simulink model "DC_motor_simulink"  (R2024b)
settings: Solver=ode45  StartTime=0.0  StopTime=2000  RelTol=1e-3
model workspace (MAT data in the model file):
  S = [0; 0; 0.05; 0; 0; -0.05; 0; 0]
values from neighbouring files (symbols this model uses):
  B = 0.81    [DC_motor_script.m]
  d = 680e-3    (= 0.68)    [DC_motor_script.m]
  E_n = Ks*Ie_r*omega_b    (= 538.36426107)    [DC_motor_script.m]
  Ie_r = 5    [DC_motor_script.m]
  J = m_max*((rho^2*d^2)/4)    (= 90.6180715851)    [DC_motor_script.m]
  Ks = 1.06    [DC_motor_script.m]
  L = [0;1;3;4;6;8;9;10]    [DC_motor_script.m]
  La = tau_a*Ra    (= 0.0039)    [DC_motor_script.m]
  Le = tau_e*Re    (= 1.2)    [DC_motor_script.m]
  m_max = mt+130*80    (= 25400)    [DC_motor_script.m]
  omega_b = 970*(2*pi/60)    (= 101.578162466)    [DC_motor_script.m]
  omega_max = (v_max/3.6)*2/(d*rho)    (= 195.32428356)    [DC_motor_script.m]
  Ra = 0.39    [DC_motor_script.m]
  Re = 12    [DC_motor_script.m]
  rho = 13/74    (= 0.175675675676)    [DC_motor_script.m]
  Tn = Pr_tot/omega_b    (= 826.949395034)    [DC_motor_script.m]
  V = [v_r/2;v_r;v_r;v_max;v_r;v_r;v_r/2;0]    [DC_motor_script.m]
  Va_r = 600    [DC_motor_script.m]
  Ve_r = 60    [DC_motor_script.m]
undefined symbols (not defined in the file or in its folder): Ccurr, Cexc_curr, Cspeed
libraries: slpidlib x3
settings Model: Creator=migli  LastModifiedBy=migli

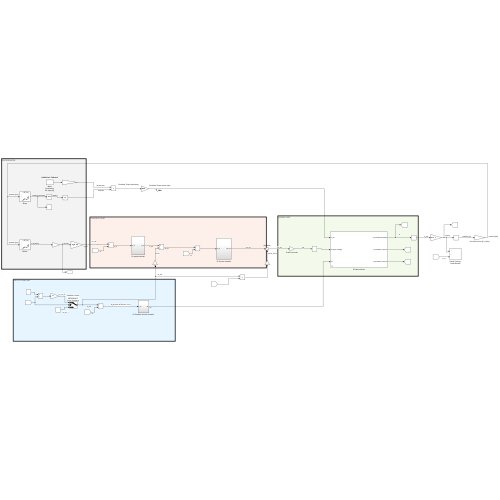
[thumbnail: Simulink's stored preview of the top-level diagram]
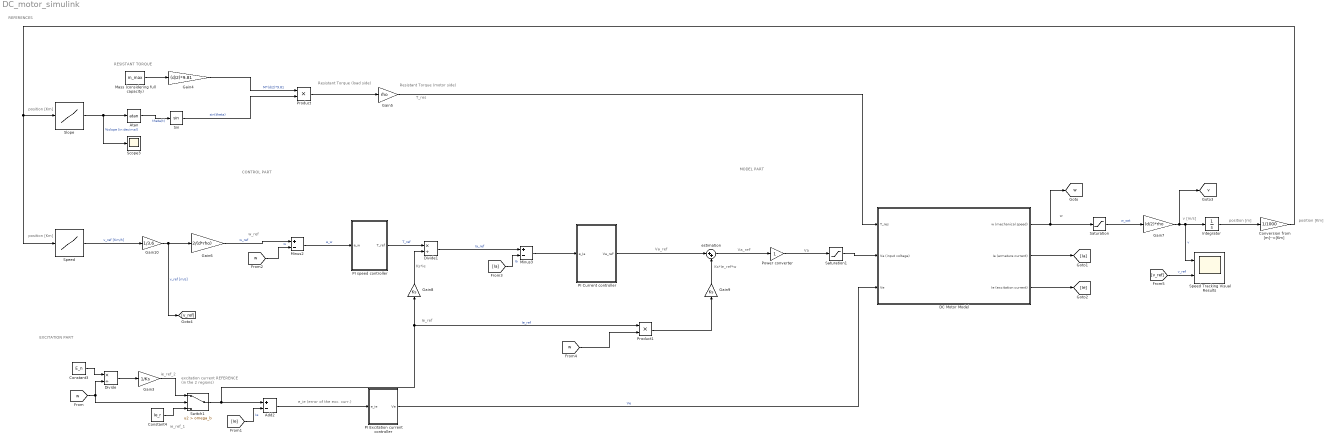
== system DC_motor_simulink ==
  note: T_res
  note: MODEL PART
  note: REFERENCES
  note: CONTROL PART
  note: EXCITATION PART
  note: position [m]
  note: e_ie (error of the exc. curr.)
  note: Va
  note: Va_ref'
  note: Va_ref
  note: Ks*ie
  note: position [Km]
  note: RESISTANT TORQUE
  note: Resistant Torque (motor side)
  note: Resistant Torque (load side)
  note: w_ref
  note: position [Km]
  note: excitation current
      |   REFERENCE
      | (in the 2 regions)
  note: ie_ref_2
  note: ie_ref_1
  note: Ie_ref
  note: Ks*Ie_ref*w
  note: position [Km]
  note: v [m/s]
  note: w
  Add2 : Sum  Inputs=+-
  Atan : Trigonometry  Operator=atan
  Constant3 : Constant  Value=E_n
  Constant4 : Constant  Value=Ie_r
  "Conversion from [m]-->[Km] " : Gain  Gain=1/1000
  DC Motor Model : Subsystem
      mask DialogControl DescTextVar Prompt: PMDC model
  Divide : Product  Inputs=*/
  Divide1 : Product  Inputs=*/
  Gain10 : Gain  Gain=1/3.6
  Gain3 : Gain  Gain=1/Ks
  Gain4 : Gain  Gain=(d/2)*9.81
  Gain5 : Gain  Gain=rho
  Gain6 : Gain  Gain=2/(d*rho)
  Gain7 : Gain  Gain=(d/2)*rho
  Gain8 : Gain  Gain=Ks
  Gain9 : Gain  Gain=Ks
  Integrator : Integrator
  Mass (considering full capacity) : Constant  Value=m_max
  Minus2 : Sum  Inputs=+-
  Minus3 : Sum  Inputs=+-
  PI Current controller : Subsystem
  PI Excitation current controller : Subsystem
  PI speed controller : Subsystem
  Power converter : Gain
  Product : Product
  Product1 : Product
  Saturation : Saturate  UpperLimit=omega_max+300  LowerLimit=0
  Saturation1 : Saturate  UpperLimit=Va_r*1000  LowerLimit=-Va_r*1000
  Scope3 : Scope
  Sin : Trigonometry
  Slope : Lookup_n-D  NumberOfTableDimensions=1  BreakpointsForDimension1=L  Table=S  InterpMethod=Flat  InternalRulePriority=Speed  RndMeth=Simplest
  Speed : Lookup_n-D  NumberOfTableDimensions=1  BreakpointsForDimension1=L  Table=V  InterpMethod=Flat  InternalRulePriority=Speed  RndMeth=Simplest
  Speed Tracking Visual Results : Scope  NumInputPorts=2
  Switch1 : Switch  Criteria=u2 > Threshold  Threshold=omega_b  SaturateOnIntegerOverflow=off  InputSameDT=off
  estimation : Sum  Inputs=|++
  tag scope: v=global, w=global
  wires:
  Atan/1 -> Sin/1  "theta(t)"
  Mass (considering full capacity)/1 -> Gain4/1
  Product/1 -> Gain5/1
  Slope/1 -> Scope3/1, Atan/1  "%slope (in decimal)"
  Sin/1 -> Product/2  "sin(theta)"
  Gain4/1 -> Product/1  "M*(d/2)*9.81"
  Speed/1 -> Gain10/1  "v_ref [Km/h]"
  Gain6/1 -> Minus2/1  "w_ref"
  [w] -> Minus2/2  "w"
  Minus2/1 -> PI speed controller/1(e_w)  "e_w"
  PI speed controller/1(T_ref) -> Divide1/1  "T_ref"
  Gain8/1 -> Divide1/2
  Gain3/1 -> Switch1/1
  Constant4/1 -> Switch1/3
  [w] -> Divide/2, Switch1/2
  Switch1/1 -> Product1/1, Gain8/1, Add2/1  "Ie_ref"
  [Ie] -> Add2/2  "Ie"
  Constant3/1 -> Divide/1
  Divide/1 -> Gain3/1
  Divide1/1 -> Minus3/1  "Ia_ref"
  [Ia] -> Minus3/2  "Ia"
  Minus3/1 -> PI Current controller/1(e_Ia)
  PI Current controller/1(Va_ref') -> estimation/1
  Gain9/1 -> estimation/2
  [w] -> Product1/2
  Product1/1 -> Gain9/1
  estimation/1 -> Power converter/1
  Power converter/1 -> Saturation1/1
  Saturation1/1 -> DC Motor Model/2(Va (input voltage))
  Gain5/1 -> DC Motor Model/1(T_res)
  Add2/1 -> PI Excitation current controller/1(e_ie)
  PI Excitation current controller/1(Ve) -> DC Motor Model/3(Ve)  "Ve"
  Gain7/1 -> [v], Speed Tracking Visual Results/1, Integrator/1  "v"
  Integrator/1 -> "Conversion from [m]-->[Km] "/1
  "Conversion from [m]-->[Km] "/1 -> Speed/1, Slope/1
  DC Motor Model/2(Ia (armature current)) -> [Ia]
  DC Motor Model/3(Ie (excitation current)) -> [Ie]
  Gain10/1 -> [v_ref], Gain6/1  "v_ref [m/s]"
  DC Motor Model/1(w (mechanical speed)) -> [w], Saturation/1
  Saturation/1 -> Gain7/1  "w_sat"
  [v_ref] -> Speed Tracking Visual Results/2  "v_ref"

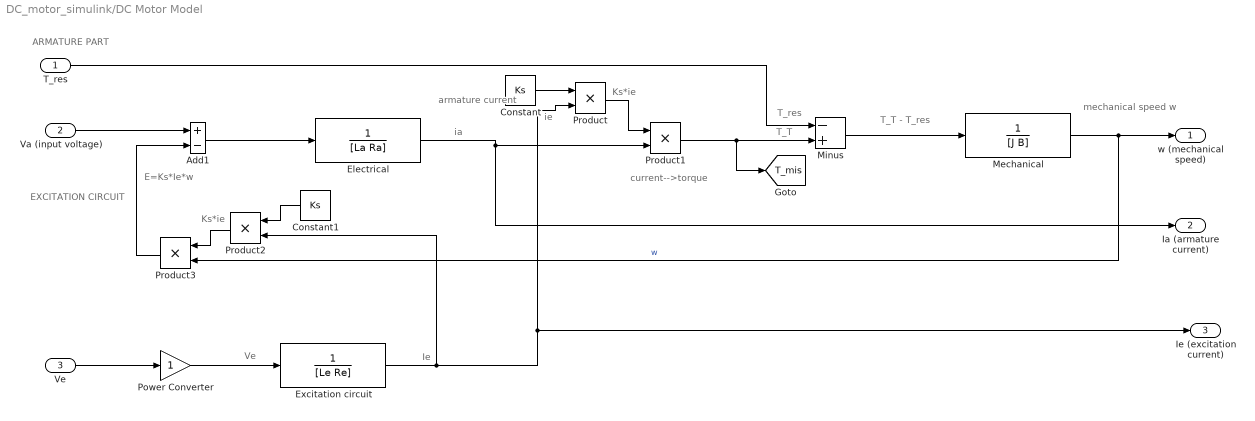
== system DC_motor_simulink/DC Motor Model ==
  note: ARMATURE PART
  note: EXCITATION CIRCUIT
  note: E=Ks*Ie*w
  note: Ks*ie
  note: current-->torque
  note: ie
  note: ia
  note: Ie
  note: Ve
  note: T_T - T_res
  note: T_res
  note: T_T
  note: mechanical speed
      |              w
  note: armature
      |  current
  note: Ks*ie
  T_res : Inport
  Va (input voltage) : Inport  Port=2
  Ve : Inport  Port=3
  Add1 : Sum  Inputs=+-
  Constant : Constant  Value=Ks
  Constant1 : Constant  Value=Ks
  Electrical : TransferFcn  Denominator=[La Ra]
  Excitation circuit : TransferFcn  Denominator=[Le Re]
  Mechanical : TransferFcn  Denominator=[J B]
  Minus : Sum  Inputs=-+
  Power Converter : Gain
  Product{,1..3} (4 alike) : Product
  w (mechanical speed) : Outport
  Ia (armature current) : Outport  Port=2
  Ie (excitation current) : Outport  Port=3
  tag scope: T_mis=global
  wires:
  Add1/1 -> Electrical/1
  Electrical/1 -> Product1/2, Ia (armature current)/1
  Va (input voltage)/1 -> Add1/1
  Mechanical/1 -> Product3/2, w (mechanical speed)/1  "w"
  Minus/1 -> Mechanical/1
  T_res/1 -> Minus/1
  Excitation circuit/1 -> Ie (excitation current)/1, Product/2, Product2/2
  Constant/1 -> Product/1
  Product/1 -> Product1/1
  Product1/1 -> [T_mis], Minus/2
  Constant1/1 -> Product2/1
  Product2/1 -> Product3/1
  Product3/1 -> Add1/2
  Ve/1 -> Power Converter/1
  Power Converter/1 -> Excitation circuit/1

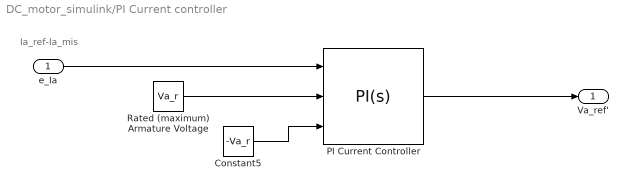
== system DC_motor_simulink/PI Current controller ==
  note: Ia_ref-Ia_mis
  e_Ia : Inport
  Constant5 : Constant  Value=-Va_r
  PI Current Controller : slpidlib/PID Controller  Controller=PI  Form=Parallel  TimeDomain=Continuous-time  UseExternalTs=off  SampleTime=-1  IntegratorMethod=Forward Euler  FilterMethod=Forward Euler  ControllerParametersSource=internal  P=Ccurr.Kp  I=Ccurr.Ki  UseKiTs=off  D=0  UseExternalDerivativeSource=off  N=100  UseFilter=on  TunerSelectOption=Transfer Function Based (PID Tuner App)  InitialConditionSource=internal  InitialConditionForIntegrator=0  InitialConditionForFilter=0  DifferentiatorICPrevScaledInput=0  ExternalReset=none  TrackingMode=off  Kt=1  LimitOutput=on  SatLimitsSource=external  UpperSaturationLimit=inf  LowerSaturationLimit=-inf  LinearizeAsGain=on  AntiWindupMode=back-calculation  Kb=Ccurr.Ki/Ccurr.Kp  LimitIntegrator=off  UpperIntegratorSaturationLimit=inf  LowerIntegratorSaturationLimit=-inf  POutMin=[]  POutMax=[]  IOutMin=[]  IOutMax=[]  DOutMin=[]  DOutMax=[]  NOutMin=[]  NOutMax=[]  SumOutMin=[]  SumOutMax=[]  SaturationOutMin=[]  SaturationOutMax=[]  PParamMin=[]  PParamMax=[]  IParamMin=[]  IParamMax=[]  DParamMin=[]  DParamMax=[]  NParamMin=[]  NParamMax=[]  KbParamMin=[]  KbParamMax=[]  KtParamMin=[]  KtParamMax=[]  KbOutMin=[]  KbOutMax=[]  KtOutMin=[]  KtOutMax=[]  IntegratorOutMin=[]  IntegratorOutMax=[]  FilterOutMin=[]  FilterOutMax=[]  SumI1OutMin=[]  SumI1OutMax=[]  SumI2OutMin=[]  SumI2OutMax=[]  SumI3OutMin=[]  SumI3OutMax=[]  SumI4OutMin=[]  SumI4OutMax=[]  SumDOutMin=[]  SumDOutMax=[]  DifferentiatorOutMin=[]  DifferentiatorOutMax=[]  FilterDiffOutCoefMin=[]  FilterDiffOutCoefMax=[]  ReciprocalOutMin=[]  ReciprocalOutMax=[]  SumDenOutMin=[]  SumDenOutMax=[]  SumNumOutMin=[]  SumNumOutMax=[]  DivideOutMin=[]  DivideOutMax=[]  UdiffTsProdOutMin=[]  UdiffTsProdOutMax=[]  NTsProdOutMin=[]  NTsProdOutMax=[]  UintegralTsProdOutMin=[]  UintegralTsProdOutMax=[]  UngainTsProdOutMin=[]  UngainTsProdOutMax=[]  ClampingZeroOutDataTypeStr=Inherit: Inherit via back propagation  ClampingZeroOutMin=[]  ClampingZeroOutMax=[]  FilterDenConstantOutDataTypeStr=Inherit: Inherit via back propagation  FilterDenConstantOutMin=[]  FilterDenConstantOutMax=[]  PCopyOutDataTypeStr=Inherit: Inherit via back propagation  PCopyOutMin=[]  PCopyOutMax=[]  NCopyOutDataTypeStr=Inherit: Inherit via back propagation  NCopyOutMin=[]  NCopyOutMax=[]  IntegratorContinuousStateAttributes=''  IntegratorStateMustResolveToSignalObject=off  IntegratorRTWStateStorageClass=Auto  FilterContinuousStateAttributes=''  FilterStateMustResolveToSignalObject=off  FilterRTWStateStorageClass=Auto  ParallelPVariant=InternalParameters  IdealPVariant=Disabled  IVariant=InternalParameters  DVariant=Disabled  IntegratorVariant=Continuous  SatVariant=External  AWVariant=BackCalculation  PCopyVariant=Disabled  TRVariant=Disabled  FdbkBlocksVariant=Forward  IdealPFdbkVariant=Disabled  SatFdbkVariant=Disabled  DerivativeFilterVariant=Disabled  NVariant=Disabled  NCopyVariant=Disabled_SignalSpec  FilterICVariant=Disabled  IntegratorICVariant=InternalICs  ExternalResetVariant=Disabled  TRSumVariant=Passthrough  SumFdbkVariant=Disabled  SumVariant=Sum_PI  TsampFilterVariant=InternalTs  TsampNgainVariant=Passthrough  TsampIntegralVariant=Disabled_SignalSpec  ExternalSaturationOutDataTypeStr=Inherit: Same as second input  DerivativeSourceVariant=Disabled  PreIntVariant=InternalPreInt
  Rated (maximum) Armature Voltage : Constant  Value=Va_r
  Va_ref' : Outport
  wires:
  e_Ia/1 -> PI Current Controller/1
  Rated (maximum) Armature Voltage/1 -> PI Current Controller/2
  Constant5/1 -> PI Current Controller/3
  PI Current Controller/1 -> Va_ref'/1

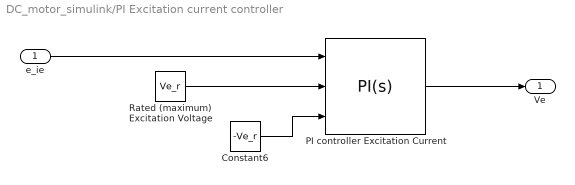
== system DC_motor_simulink/PI Excitation current controller ==
  e_ie : Inport
  Constant6 : Constant  Value=-Ve_r
  "PI controller Excitation Current " : slpidlib/PID Controller  Controller=PI  Form=Parallel  TimeDomain=Continuous-time  UseExternalTs=off  SampleTime=-1  IntegratorMethod=Forward Euler  FilterMethod=Forward Euler  ControllerParametersSource=internal  P=Cexc_curr.Kp  I=Cexc_curr.Ki  UseKiTs=off  D=0  UseExternalDerivativeSource=off  N=100  UseFilter=on  TunerSelectOption=Transfer Function Based (PID Tuner App)  InitialConditionSource=internal  InitialConditionForIntegrator=0  InitialConditionForFilter=0  DifferentiatorICPrevScaledInput=0  ExternalReset=none  TrackingMode=off  Kt=1  LimitOutput=on  SatLimitsSource=external  UpperSaturationLimit=inf  LowerSaturationLimit=-inf  LinearizeAsGain=on  AntiWindupMode=back-calculation  Kb=Cexc_curr.Ki/Cexc_curr.Kp  LimitIntegrator=off  UpperIntegratorSaturationLimit=inf  LowerIntegratorSaturationLimit=-inf  POutMin=[]  POutMax=[]  IOutMin=[]  IOutMax=[]  DOutMin=[]  DOutMax=[]  NOutMin=[]  NOutMax=[]  SumOutMin=[]  SumOutMax=[]  SaturationOutMin=[]  SaturationOutMax=[]  PParamMin=[]  PParamMax=[]  IParamMin=[]  IParamMax=[]  DParamMin=[]  DParamMax=[]  NParamMin=[]  NParamMax=[]  KbParamMin=[]  KbParamMax=[]  KtParamMin=[]  KtParamMax=[]  KbOutMin=[]  KbOutMax=[]  KtOutMin=[]  KtOutMax=[]  IntegratorOutMin=[]  IntegratorOutMax=[]  FilterOutMin=[]  FilterOutMax=[]  SumI1OutMin=[]  SumI1OutMax=[]  SumI2OutMin=[]  SumI2OutMax=[]  SumI3OutMin=[]  SumI3OutMax=[]  SumI4OutMin=[]  SumI4OutMax=[]  SumDOutMin=[]  SumDOutMax=[]  DifferentiatorOutMin=[]  DifferentiatorOutMax=[]  FilterDiffOutCoefMin=[]  FilterDiffOutCoefMax=[]  ReciprocalOutMin=[]  ReciprocalOutMax=[]  SumDenOutMin=[]  SumDenOutMax=[]  SumNumOutMin=[]  SumNumOutMax=[]  DivideOutMin=[]  DivideOutMax=[]  UdiffTsProdOutMin=[]  UdiffTsProdOutMax=[]  NTsProdOutMin=[]  NTsProdOutMax=[]  UintegralTsProdOutMin=[]  UintegralTsProdOutMax=[]  UngainTsProdOutMin=[]  UngainTsProdOutMax=[]  ClampingZeroOutDataTypeStr=Inherit: Inherit via back propagation  ClampingZeroOutMin=[]  ClampingZeroOutMax=[]  FilterDenConstantOutDataTypeStr=Inherit: Inherit via back propagation  FilterDenConstantOutMin=[]  FilterDenConstantOutMax=[]  PCopyOutDataTypeStr=Inherit: Inherit via back propagation  PCopyOutMin=[]  PCopyOutMax=[]  NCopyOutDataTypeStr=Inherit: Inherit via back propagation  NCopyOutMin=[]  NCopyOutMax=[]  IntegratorContinuousStateAttributes=''  IntegratorStateMustResolveToSignalObject=off  IntegratorRTWStateStorageClass=Auto  FilterContinuousStateAttributes=''  FilterStateMustResolveToSignalObject=off  FilterRTWStateStorageClass=Auto  ParallelPVariant=InternalParameters  IdealPVariant=Disabled  IVariant=InternalParameters  DVariant=Disabled  IntegratorVariant=Continuous  SatVariant=External  AWVariant=BackCalculation  PCopyVariant=Disabled  TRVariant=Disabled  FdbkBlocksVariant=Forward  IdealPFdbkVariant=Disabled  SatFdbkVariant=Disabled  DerivativeFilterVariant=Disabled  NVariant=Disabled  NCopyVariant=Disabled_SignalSpec  FilterICVariant=Disabled  IntegratorICVariant=InternalICs  ExternalResetVariant=Disabled  TRSumVariant=Passthrough  SumFdbkVariant=Disabled  SumVariant=Sum_PI  TsampFilterVariant=InternalTs  TsampNgainVariant=Passthrough  TsampIntegralVariant=Disabled_SignalSpec  ExternalSaturationOutDataTypeStr=Inherit: Same as second input  DerivativeSourceVariant=Disabled  PreIntVariant=InternalPreInt
  Rated (maximum) Excitation Voltage : Constant  Value=Ve_r
  Ve : Outport
  wires:
  e_ie/1 -> "PI controller Excitation Current "/1
  Constant6/1 -> "PI controller Excitation Current "/3
  Rated (maximum) Excitation Voltage/1 -> "PI controller Excitation Current "/2
  "PI controller Excitation Current "/1 -> Ve/1

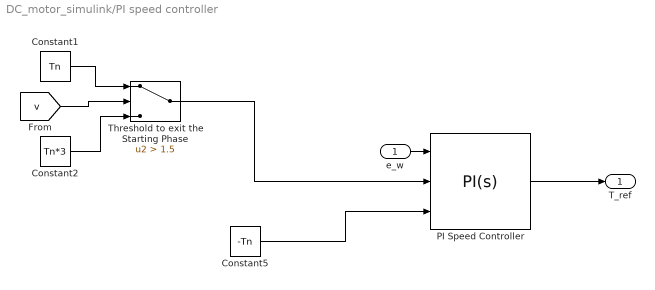
== system DC_motor_simulink/PI speed controller ==
  e_w : Inport
  Constant1 : Constant  Value=Tn
  Constant2 : Constant  Value=Tn*3
  Constant5 : Constant  Value=-Tn
  PI Speed Controller : slpidlib/PID Controller  Controller=PI  Form=Parallel  TimeDomain=Continuous-time  UseExternalTs=off  SampleTime=-1  IntegratorMethod=Forward Euler  FilterMethod=Forward Euler  ControllerParametersSource=internal  P=Cspeed.Kp  I=Cspeed.Ki  UseKiTs=off  D=0  UseExternalDerivativeSource=off  N=100  UseFilter=on  TunerSelectOption=Transfer Function Based (PID Tuner App)  InitialConditionSource=internal  InitialConditionForIntegrator=0  InitialConditionForFilter=0  DifferentiatorICPrevScaledInput=0  ExternalReset=none  TrackingMode=off  Kt=1  LimitOutput=on  SatLimitsSource=external  UpperSaturationLimit=inf  LowerSaturationLimit=-inf  LinearizeAsGain=on  AntiWindupMode=back-calculation  Kb=Cspeed.Ki/Cspeed.Kp  LimitIntegrator=off  UpperIntegratorSaturationLimit=inf  LowerIntegratorSaturationLimit=-inf  POutMin=[]  POutMax=[]  IOutMin=[]  IOutMax=[]  DOutMin=[]  DOutMax=[]  NOutMin=[]  NOutMax=[]  SumOutMin=[]  SumOutMax=[]  SaturationOutMin=[]  SaturationOutMax=[]  PParamMin=[]  PParamMax=[]  IParamMin=[]  IParamMax=[]  DParamMin=[]  DParamMax=[]  NParamMin=[]  NParamMax=[]  KbParamMin=[]  KbParamMax=[]  KtParamMin=[]  KtParamMax=[]  KbOutMin=[]  KbOutMax=[]  KtOutMin=[]  KtOutMax=[]  IntegratorOutMin=[]  IntegratorOutMax=[]  FilterOutMin=[]  FilterOutMax=[]  SumI1OutMin=[]  SumI1OutMax=[]  SumI2OutMin=[]  SumI2OutMax=[]  SumI3OutMin=[]  SumI3OutMax=[]  SumI4OutMin=[]  SumI4OutMax=[]  SumDOutMin=[]  SumDOutMax=[]  DifferentiatorOutMin=[]  DifferentiatorOutMax=[]  FilterDiffOutCoefMin=[]  FilterDiffOutCoefMax=[]  ReciprocalOutMin=[]  ReciprocalOutMax=[]  SumDenOutMin=[]  SumDenOutMax=[]  SumNumOutMin=[]  SumNumOutMax=[]  DivideOutMin=[]  DivideOutMax=[]  UdiffTsProdOutMin=[]  UdiffTsProdOutMax=[]  NTsProdOutMin=[]  NTsProdOutMax=[]  UintegralTsProdOutMin=[]  UintegralTsProdOutMax=[]  UngainTsProdOutMin=[]  UngainTsProdOutMax=[]  ClampingZeroOutDataTypeStr=Inherit: Inherit via back propagation  ClampingZeroOutMin=[]  ClampingZeroOutMax=[]  FilterDenConstantOutDataTypeStr=Inherit: Inherit via back propagation  FilterDenConstantOutMin=[]  FilterDenConstantOutMax=[]  PCopyOutDataTypeStr=Inherit: Inherit via back propagation  PCopyOutMin=[]  PCopyOutMax=[]  NCopyOutDataTypeStr=Inherit: Inherit via back propagation  NCopyOutMin=[]  NCopyOutMax=[]  IntegratorContinuousStateAttributes=''  IntegratorStateMustResolveToSignalObject=off  IntegratorRTWStateStorageClass=Auto  FilterContinuousStateAttributes=''  FilterStateMustResolveToSignalObject=off  FilterRTWStateStorageClass=Auto  ParallelPVariant=InternalParameters  IdealPVariant=Disabled  IVariant=InternalParameters  DVariant=Disabled  IntegratorVariant=Continuous  SatVariant=External  AWVariant=BackCalculation  PCopyVariant=Disabled  TRVariant=Disabled  FdbkBlocksVariant=Forward  IdealPFdbkVariant=Disabled  SatFdbkVariant=Disabled  DerivativeFilterVariant=Disabled  NVariant=Disabled  NCopyVariant=Disabled_SignalSpec  FilterICVariant=Disabled  IntegratorICVariant=InternalICs  ExternalResetVariant=Disabled  TRSumVariant=Passthrough  SumFdbkVariant=Disabled  SumVariant=Sum_PI  TsampFilterVariant=InternalTs  TsampNgainVariant=Passthrough  TsampIntegralVariant=Disabled_SignalSpec  ExternalSaturationOutDataTypeStr=Inherit: Same as second input  DerivativeSourceVariant=Disabled  PreIntVariant=InternalPreInt
  Threshold to exit the Starting Phase : Switch  Criteria=u2 > Threshold  Threshold=1.5  SaturateOnIntegerOverflow=off  InputSameDT=off
  T_ref : Outport
  wires:
  Constant2/1 -> Threshold to exit the Starting Phase/3
  PI Speed Controller/1 -> T_ref/1
  Constant1/1 -> Threshold to exit the Starting Phase/1
  e_w/1 -> PI Speed Controller/1
  [v] -> Threshold to exit the Starting Phase/2
  Threshold to exit the Starting Phase/1 -> PI Speed Controller/2
  Constant5/1 -> PI Speed Controller/3
